simulink model "Robot"  (Simulink 7.2)
settings: Solver=ode45  StartTime=0.0  StopTime=2.0  RelTol=1e-3
settings Model: Creator=reynaud  LastModifiedBy=reynaud
settings DebuggingCC: AlgebraicLoopMsg=none  SolverPrmCheckMsg=none  UnconnectedInputMsg=none  UnconnectedOutputMsg=none  UnconnectedLineMsg=none

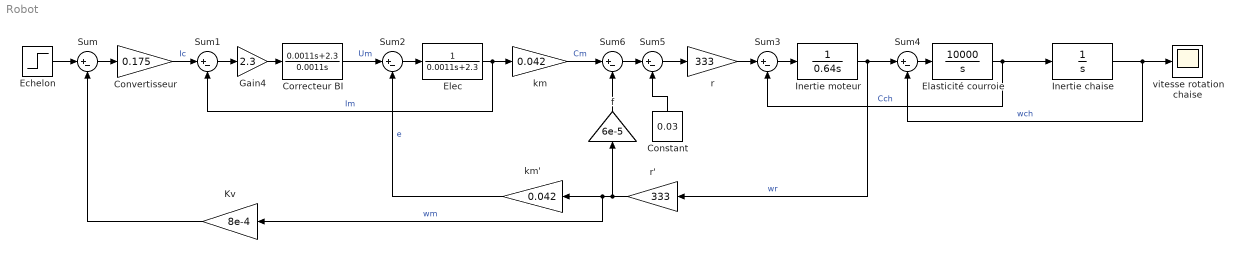
== system Robot ==
  Constant : Constant  Orientation=up  Value=0.03  OutDataType=sfix(16)  OutScaling=2^0
  Convertisseur : Gain  Gain=0.175  ParameterDataType=sfix(16)  ParameterScaling=2^0  OutDataType=sfix(16)  OutScaling=2^0
  Correcteur BI : TransferFcn  Numerator=[0.0011,2.3]  Denominator=[0.0011 0]
  Echelon : Step  Time=0  After=10  SampleTime=0
  Elasticité courroie : TransferFcn  Numerator=[10000]  Denominator=[1 0]
  Elec : TransferFcn  Denominator=[0.0011 2.3]
  Gain4 : Gain  Gain=2.3  ParameterDataType=sfix(16)  ParameterScaling=2^0  OutDataType=sfix(16)  OutScaling=2^0
  Inertie chaise : TransferFcn  Denominator=[1 0]
  Inertie moteur : TransferFcn  Denominator=[0.64 0]
  Kv : Gain  Orientation=left  Gain=8e-4  ParameterDataType=sfix(16)  ParameterScaling=2^0  OutDataType=sfix(16)  OutScaling=2^0
  Sum{,1..6} (7 alike) : Sum  Inputs=|+-  OutDataType=sfix(16)  OutScaling=2^0
  f : Gain  Orientation=up  Gain=6e-5  ParameterDataType=sfix(16)  ParameterScaling=2^0  OutDataType=sfix(16)  OutScaling=2^0
  km : Gain  Gain=0.042  ParameterDataType=sfix(16)  ParameterScaling=2^0  OutDataType=sfix(16)  OutScaling=2^0
  km' : Gain  Orientation=left  Gain=0.042  ParameterDataType=sfix(16)  ParameterScaling=2^0  OutDataType=sfix(16)  OutScaling=2^0
  r : Gain  Gain=333  ParameterDataType=sfix(16)  ParameterScaling=2^0  OutDataType=sfix(16)  OutScaling=2^0
  r' : Gain  Orientation=left  Gain=333  ParameterDataType=sfix(16)  ParameterScaling=2^0  OutDataType=sfix(16)  OutScaling=2^0
  vitesse rotation chaise : Scope
      settings: SaveName=vitesse_rotation  DataFormat=Array
  wires:
  Echelon/1 -> Sum/1
  Sum/1 -> Convertisseur/1
  Convertisseur/1 -> Sum1/1  "Ic"
  Correcteur BI/1 -> Sum2/1  "Um"
  Sum2/1 -> Elec/1
  Elec/1 -> Sum1/2, km/1  "Im"
  r/1 -> Sum3/1
  Inertie moteur/1 -> Sum4/1, r'/1  "wr"
  Sum4/1 -> Elasticité courroie/1
  Elasticité courroie/1 -> Sum3/2, Inertie chaise/1  "Cch"
  Inertie chaise/1 -> Sum4/2, vitesse rotation chaise/1  "wch"
  km'/1 -> Sum2/2  "e"
  Sum1/1 -> Gain4/1
  Gain4/1 -> Correcteur BI/1
  Sum3/1 -> Inertie moteur/1
  Kv/1 -> Sum/2
  r'/1 -> km'/1, Kv/1, f/1  "wm"
  km/1 -> Sum6/1  "Cm"
  f/1 -> Sum6/2
  Sum6/1 -> Sum5/1
  Sum5/1 -> r/1
  Constant/1 -> Sum5/2
